simulink model "Lead2AxisController"  (R2024a)
settings: Solver=VariableStepAuto  StartTime=0.0  StopTime=10.0  RelTol=1e-3
values from neighbouring files (symbols this model uses):
  integrateblk_x_z = c2d(integrateblk_x,Ts)    [ControllerSetupFunction.m]
  integrateblk_y_z = c2d(integrateblk_y,Ts)    [ControllerSetupFunction.m]
  Ka = 1    [ControllerSetupFunction.m]
  Kd = 1    [ControllerSetupFunction.m]
  Kt = 0.49    [ControllerSetupFunction.m]
  LeadComp_x_z = c2d(LeadComp_x,Ts)    [ControllerSetupFunction.m]
  LeadComp_y_z = c2d(LeadComp_y,Ts)    [ControllerSetupFunction.m]
  Ts = 0.0001    [ControllerSetupFunction.m]
libraries: cstblocks x6
settings Model: Creator=bobsy  LastModifiedBy=bobsy

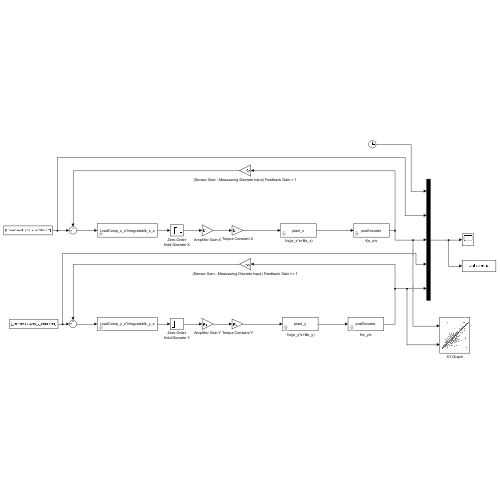
[thumbnail: Simulink's stored preview of the top-level diagram]
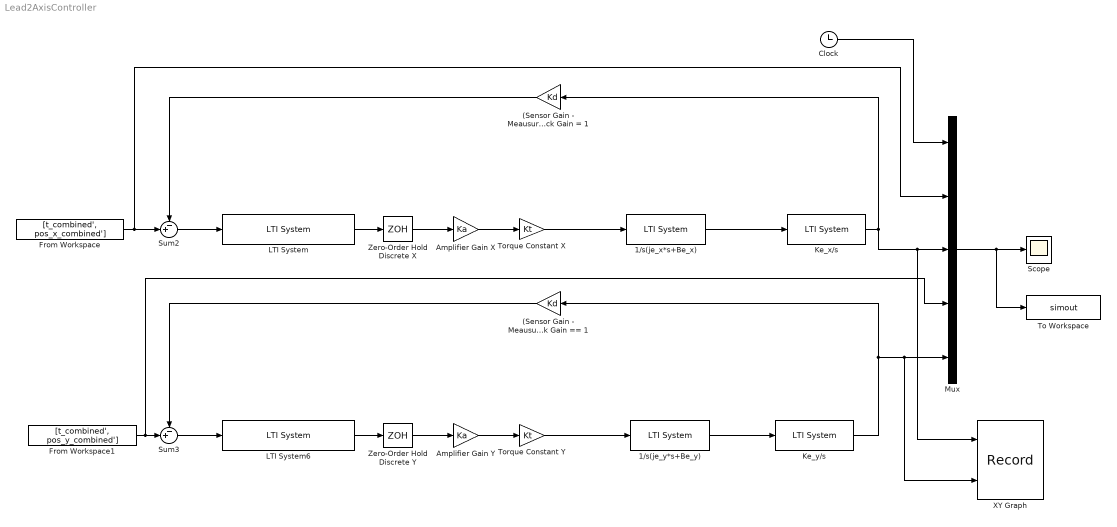
== system Lead2AxisController ==
  (Sensor Gain - Meausuring Discrete Input) Feedback Gain = 1 : Gain  Gain=Kd
  (Sensor Gain - Meausuring Discrete Input) Feedback Gain == 1 : Gain  Gain=Kd
  1/s(je_x*s+Be_x) : cstblocks/LTI System  sys=plant_x  IC=[]  PadeOrder=0
  1/s(je_y*s+Be_y) : cstblocks/LTI System  sys=plant_y  IC=[]  PadeOrder=0
  Amplifier Gain X : Gain  Gain=Ka
  Amplifier Gain Y : Gain  Gain=Ka
  Clock : Clock
  From Workspace : FromWorkspace  VariableName=[t_combined', pos_x_combined']
  From Workspace1 : FromWorkspace  VariableName=[t_combined', pos_y_combined']
  Ke_x/s : cstblocks/LTI System  sys=posEncoder  IC=[]  PadeOrder=0
  Ke_y/s : cstblocks/LTI System  sys=posEncoder  IC=[]  PadeOrder=0
  LTI System : cstblocks/LTI System  sys=LeadComp_x_z*integrateblk_x_z  IC=[]  PadeOrder=0
  LTI System6 : cstblocks/LTI System  sys=LeadComp_y_z*integrateblk_y_z  IC=[]  PadeOrder=0
  Mux : Mux  Inputs=5
  Scope : Scope
  Sum2 : Sum  Inputs=-+|
  Sum3 : Sum  Inputs=-+|
  To Workspace : ToWorkspace  VariableName=simout  SaveFormat=Timeseries  SampleTime=-1
  Torque Constant X : Gain  Gain=Kt
  Torque Constant Y : Gain  Gain=Kt
  XY Graph : Record  FileSettingsInternal="{\"entries\":[{\"content\":{\"excelSettings\":{\"content\":{},\"type\":\"Streamout.ExcelSettings\"}},\"type\":\"Streamout.FileSettingStorage\",\"uuid\":\"\"}],\"packageUris\":[\"http:\\/\\/schema.mathworks.com\\/mf0\\/streamout_blocks\\/R2020a\"],\"version\":\"1.0\"}"  Layout=[1 1]  SignalsInternal="{\"entries\":[{\"content\":{\"signals\":[{\"content\":{\"blockPath\":[],\"dimensions\":[1],\"domain\":\"\",\"lineColor\":\"#a2142f\",\"plots\":[ 1 ],\"port\":1,\"sid\":[\"\"],\"signalID\":1,\"signalName\":\"Ke_x\\/s\"},\"type\":\"RecordBlkView.Signal\",\"uuid\":\"\"},{\"content\":{\"blockPath\":[],\"dimensions\":[1],\"domain\":\"\",\"lineColor\":\"#139fff\",\"plots\":[ 1 ],\"port\":2,\"sid\":[\"\"],\"signalID\":2,\"signalName\":\"Ke_y\\/s\"},\"type\":\"RecordBlkView.Signal\",\"uuid\":\"\"}]},\"type\":\"RecordBlkView.InputSignals\",\"uuid\":\"\"}],\"packageUris\":[\"http:\\/\\/schema.mathworks.com\\/mf0\\/streamout_blocks\\/R2020a\"],\"version\":\"1.0\"}"  VisualizationBindings="{\"xyplotplugin\":{\"info\":[{\"series\":[{\"bindingParametersList\":[{\"parameter\":\"X-Axis\",\"signalID\":1,\"signalName\":\"Ke_x\\/s\"},{\"parameter\":\"Y-Axis\",\"signalID\":2,\"signalName\":\"Ke_y\\/s\"}],\"seriesID\":0}],\"subplotID\":1}]}}"  CompatibilityTag=XY
  Zero-Order Hold Discrete X : ZeroOrderHold  SampleTime=Ts
  Zero-Order Hold Discrete Y : ZeroOrderHold  SampleTime=Ts
  wires:
  Ke_x/s/1 -> (Sensor Gain - Meausuring Discrete Input) Feedback Gain = 1/1, XY Graph/1, Mux/3
  (Sensor Gain - Meausuring Discrete Input) Feedback Gain = 1/1 -> Sum2/1
  Sum2/1 -> LTI System/1
  Zero-Order Hold Discrete X/1 -> Amplifier Gain X/1
  LTI System/1 -> Zero-Order Hold Discrete X/1
  Torque Constant X/1 -> 1/s(je_x*s+Be_x)/1
  1/s(je_x*s+Be_x)/1 -> Ke_x/s/1
  Amplifier Gain X/1 -> Torque Constant X/1
  Sum3/1 -> LTI System6/1
  1/s(je_y*s+Be_y)/1 -> Ke_y/s/1
  (Sensor Gain - Meausuring Discrete Input) Feedback Gain == 1/1 -> Sum3/1
  Ke_y/s/1 -> (Sensor Gain - Meausuring Discrete Input) Feedback Gain == 1/1, XY Graph/2, Mux/5
  Torque Constant Y/1 -> 1/s(je_y*s+Be_y)/1
  Amplifier Gain Y/1 -> Torque Constant Y/1
  Zero-Order Hold Discrete Y/1 -> Amplifier Gain Y/1
  LTI System6/1 -> Zero-Order Hold Discrete Y/1
  From Workspace/1 -> Mux/2, Sum2/2
  From Workspace1/1 -> Mux/4, Sum3/2
  Clock/1 -> Mux/1
  Mux/1 -> To Workspace/1, Scope/1
